simulink model "two_area_model_PI_control"  (R2014b)
settings: Solver=ode4  StartTime=0.0  StopTime=30.0  FixedStep=0.01  RelTol=1e-3
settings Model: Creator=Shane Reynolds  LastModifiedBy=Shane Reynolds

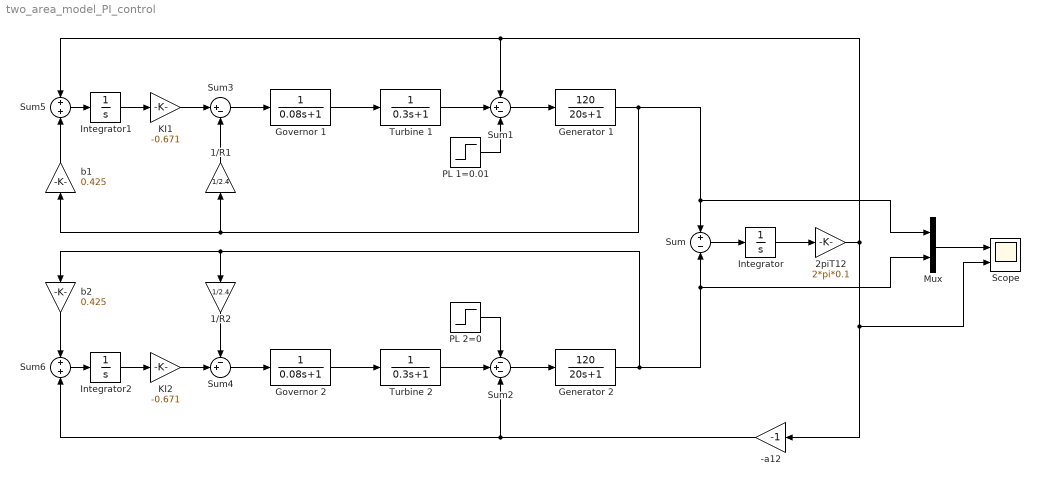
== system two_area_model_PI_control ==
  -a12 : Gain  Gain=-1
  1/R1 : Gain  Gain=1/2.4
  1/R2 : Gain  Gain=1/2.4
  2piT12 : Gain  Gain=2*pi*0.1
  Generator 1 : TransferFcn  Numerator=[120]  Denominator=[20 1]
  Generator 2 : TransferFcn  Numerator=[120]  Denominator=[20 1]
  Governor 1 : TransferFcn  Denominator=[0.08 1]
  Governor 2 : TransferFcn  Denominator=[0.08 1]
  Integrator : Integrator
  Integrator1 : Integrator
  Integrator2 : Integrator
  KI1 : Gain  Gain=-0.671
  KI2 : Gain  Gain=-0.671
  Mux : Mux  Inputs=2
  PL 1=0.01 : Step  After=0.01  SampleTime=0
  PL 2=0 : Step  After=0  SampleTime=0
  Scope : Scope  NumInputPorts=2
      settings: YMin=-5~-5  YMax=5~5
  Sum : Sum  Inputs=+|-
  Sum1 : Sum  Inputs=-+-
  Sum2 : Sum  Inputs=-+-
  Sum3 : Sum  Inputs=|+-
  Sum4 : Sum  Inputs=-+|
  Sum5 : Sum  Inputs=+|+
  Sum6 : Sum  Inputs=+|+
  Turbine 1 : TransferFcn  Denominator=[0.3 1]
  Turbine 2 : TransferFcn  Denominator=[0.3 1]
  b1 : Gain  Gain=0.425
  b2 : Gain  Gain=0.425
  wires:
  Turbine 1/1 -> Sum1/2
  Sum1/1 -> Generator 1/1
  Turbine 2/1 -> Sum2/2
  Sum2/1 -> Generator 2/1
  Governor 1/1 -> Turbine 1/1
  Governor 2/1 -> Turbine 2/1
  Sum4/1 -> Governor 2/1
  Sum3/1 -> Governor 1/1
  Generator 1/1 -> Sum/1, Mux/1, b1/1, 1/R1/1
  Generator 2/1 -> Sum/2, Mux/2, 1/R2/1, b2/1
  Sum/1 -> Integrator/1
  Integrator/1 -> 2piT12/1
  1/R1/1 -> Sum3/2
  1/R2/1 -> Sum4/1
  2piT12/1 -> Scope/2, -a12/1, Sum5/1, Sum1/1
  -a12/1 -> Sum2/3, Sum6/2
  Mux/1 -> Scope/1
  PL 1=0.01/1 -> Sum1/3
  PL 2=0/1 -> Sum2/1
  b1/1 -> Sum5/2
  Integrator1/1 -> KI1/1
  Integrator2/1 -> KI2/1
  KI1/1 -> Sum3/1
  KI2/1 -> Sum4/2
  Sum5/1 -> Integrator1/1
  Sum6/1 -> Integrator2/1
  b2/1 -> Sum6/1
